simulink model "Pneumatic_System"  (R2016b)
settings: Solver=FixedStepDiscrete  StartTime=0.0  StopTime=inf  FixedStep=PnmSys.tiSimnTiStep_C  RelTol=1e-3  EnableMultiTasking=on
settings Model: Creator=djuenema  LastModifiedBy=djuenema
settings DataIOCC: SaveFormat=StructureWithTime  SaveOutput=off  DSMLogging=off  VisualizeSimOutput=off  SaveTime=off  SignalLoggingName=Results
settings OptimizationCC: BlockReduction=off  ConditionallyExecuteInputs=off  LifeSpan=inf
settings DebuggingCC: AllowSymbolicDim=off  SFUnexpectedBacktrackingDiag=warning  SFNoUnconditionalDefaultTransitionDiag=warning  SFExecutionAtInitializationDiag=none
settings ModelReferenceCC: ModelReferenceNumInstancesAllowed=Single  PropagateSignalLabelsOutOfModel=off
settings GRTTargetCC: TargetLangStandard=C89/C90 (ANSI)
settings ConfigComp: CovMetricSettings=dw  CovHtmlReporting=on  CovSaveCumulativeToWorkspaceVar=on  CovSaveSingleToWorkspaceVar=on  CovExternalEMLEnable=off

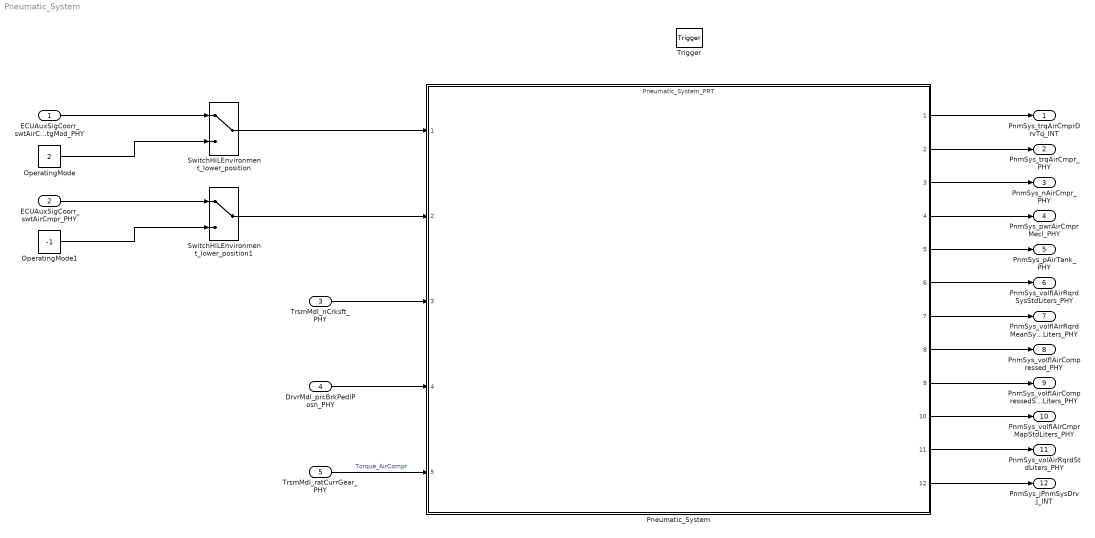
== system Pneumatic_System ==
  ECUAuxSigCoorr_swtAirCmprOpertgMod_PHY : Inport
  ECUAuxSigCoorr_swtAirCmpr_PHY : Inport  Port=2
  TrsmMdl_nCrksft_PHY : Inport  Port=3
  DrvrMdl_prcBrkPedlPosn_PHY : Inport  Port=4
  TrsmMdl_ratCurrGear_PHY : Inport  Port=5
  Trigger : TriggerPort  TriggerType=function-call  VariantControl=Variant  PortDimensions=1
  OperatingMode : Constant  Value=2
  OperatingMode1 : Constant  Value=-1
  Pneumatic_System : ModelReference  ModelNameDialog=Pneumatic_System_PRT.slxp  ModelReferenceVersion=1.3  CopyOfModelProtected=on
  SwitchHiLEnvironment_lower_position : ManualSwitch
  SwitchHiLEnvironment_lower_position1 : ManualSwitch
  PnmSys_trqAirCmprDrvTq_INT : Outport
  PnmSys_trqAirCmpr_PHY : Outport  Port=2
  PnmSys_nAirCmpr_PHY : Outport  Port=3
  PnmSys_pwrAirCmprMecl_PHY : Outport  Port=4
  PnmSys_pAirTank_PHY : Outport  Port=5
  PnmSys_volflAirRqrdSysStdLiters_PHY : Outport  Port=6
  PnmSys_volflAirRqrdMeanSysStdLiters_PHY : Outport  Port=7
  PnmSys_volflAirCompressed_PHY : Outport  Port=8
  PnmSys_volflAirCompressedStdLiters_PHY : Outport  Port=9
  PnmSys_volflAirCmprMapStdLiters_PHY : Outport  Port=10
  PnmSys_volAirRqrdStdLiters_PHY : Outport  Port=11
  PnmSys_jPnmSysDrvJ_INT : Outport  Port=12
  wires:
  ECUAuxSigCoorr_swtAirCmprOpertgMod_PHY/1 -> SwitchHiLEnvironment_lower_position/1
  ECUAuxSigCoorr_swtAirCmpr_PHY/1 -> SwitchHiLEnvironment_lower_position1/1
  TrsmMdl_nCrksft_PHY/1 -> Pneumatic_System/3
  DrvrMdl_prcBrkPedlPosn_PHY/1 -> Pneumatic_System/4
  TrsmMdl_ratCurrGear_PHY/1 -> Pneumatic_System/5  "Torque_AirCompr"
  Pneumatic_System/1 -> PnmSys_trqAirCmprDrvTq_INT/1
  Pneumatic_System/2 -> PnmSys_trqAirCmpr_PHY/1
  Pneumatic_System/3 -> PnmSys_nAirCmpr_PHY/1
  Pneumatic_System/4 -> PnmSys_pwrAirCmprMecl_PHY/1
  Pneumatic_System/5 -> PnmSys_pAirTank_PHY/1
  Pneumatic_System/6 -> PnmSys_volflAirRqrdSysStdLiters_PHY/1
  Pneumatic_System/7 -> PnmSys_volflAirRqrdMeanSysStdLiters_PHY/1
  Pneumatic_System/8 -> PnmSys_volflAirCompressed_PHY/1
  Pneumatic_System/9 -> PnmSys_volflAirCompressedStdLiters_PHY/1
  Pneumatic_System/10 -> PnmSys_volflAirCmprMapStdLiters_PHY/1
  Pneumatic_System/11 -> PnmSys_volAirRqrdStdLiters_PHY/1
  Pneumatic_System/12 -> PnmSys_jPnmSysDrvJ_INT/1
  OperatingMode/1 -> SwitchHiLEnvironment_lower_position/2
  SwitchHiLEnvironment_lower_position/1 -> Pneumatic_System/1
  OperatingMode1/1 -> SwitchHiLEnvironment_lower_position1/2
  SwitchHiLEnvironment_lower_position1/1 -> Pneumatic_System/2
